simulink model "SPGF_FSK_0000_R2022b"  (R2022b)
settings: Solver=ode4  StartTime=0.0  StopTime=1.4  FixedStep=50e-6/50  RelTol=1e-3  EnableMultiTasking=on
undefined symbols (not defined in the file): D11, Delta
libraries: spsSeriesRLCBranchLib x1646, spsGroundLib x360, spsStairGeneratorLib x147, spsIdealSwitchLib x145, spsCurrentMeasurementLib x145, spsUniversalBridgeLib x76, spsThreePhaseSeriesRLCLoadLib x57, simulink x45, spsBistableLib x36, spsSequenceAnalyzerLib x31, spsThreePhaseParallelRLCLoadLib x20, spsThreePhaseTransformerTwoWindingsLib x20
(part 1 of 40)
settings Model: SimulationMode=accelerator  Creator=Anastasia  LastModifiedBy=Fedot
settings SolverCC: AlgebraicLoopSolver=TrustRegion
settings DataIOCC: SaveFormat=Array  SaveOutput=off  SignalLogging=off  DSMLogging=off  SaveTime=off  ReturnWorkspaceOutputs=off
settings OptimizationCC: BlockReduction=off  OptimizeBlockIOStorage=off  BufferReuse=off  GlobalBufferReuse=off  ExpressionFolding=off  LocalBlockOutputs=off  EfficientMapNaN2IntZero=off  LifeSpan=inf
settings DebuggingCC: UnderspecifiedInitializationDetection=Classic  MergeDetectMultiDrivingBlocksExec=none  SolverPrmCheckMsg=warning  AllowSymbolicDim=off  StateNameClashWarn=warning  SFUnexpectedBacktrackingDiag=warning  SFNoUnconditionalDefaultTransitionDiag=warning  SFExecutionAtInitializationDiag=none  SFMachineParentedDataDiag=warning  ArithmeticOperatorsInVariantConditions=warning
settings HardwareCC: ProdBitPerPointer=32  ProdBitPerSizeT=32  ProdBitPerPtrDiffT=32  ProdLargestAtomicFloat=None  ProdIntDivRoundTo=Undefined  ProdEndianess=Unspecified  ProdWordSize=32  ProdHWDeviceType=32-bit Generic  TargetBitPerPointer=64  TargetBitPerSizeT=64  TargetBitPerPtrDiffT=64  TargetLongLongMode=on  TargetIntDivRoundTo=Zero  TargetEndianess=LittleEndian  TargetWordSize=64  TargetHWDeviceType=MATLAB Host  ProdEqTarget=off
settings ModelReferenceCC: EnableRefExpFcnMdlSchedulingChecks=on  PropagateSignalLabelsOutOfModel=off
settings SFSimCC: SimUseLocalCustomCode=off  CustomCodeUndefinedFunction=UseInterfaceOnly
settings RTWCC: RTWUseLocalCustomCode=off
settings CodeAppCC: MaxIdLength=128  StateflowObjectComments=on
settings GRTTargetCC: TargetLangStandard=C89/C90 (ANSI)  CombineOutputUpdateFcns=off  GRTInterface=on
settings ConfigComp: CovMetricSettings=dw  CovSaveCumulativeToWorkspaceVar=on  CovSaveSingleToWorkspaceVar=on  CovExternalEMLEnable=off
settings SimscapeCC: SimscapeNormalizeSystem=off

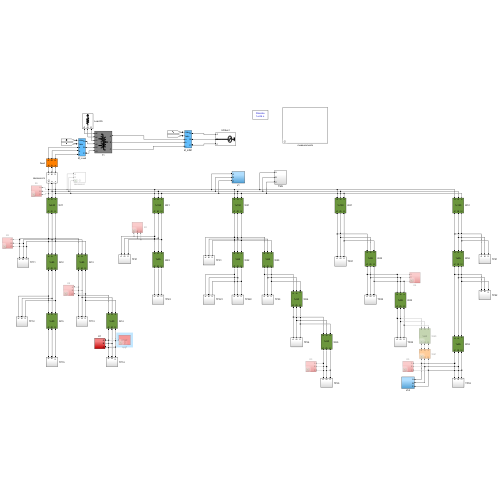
[thumbnail: Simulink's stored preview of the top-level diagram]
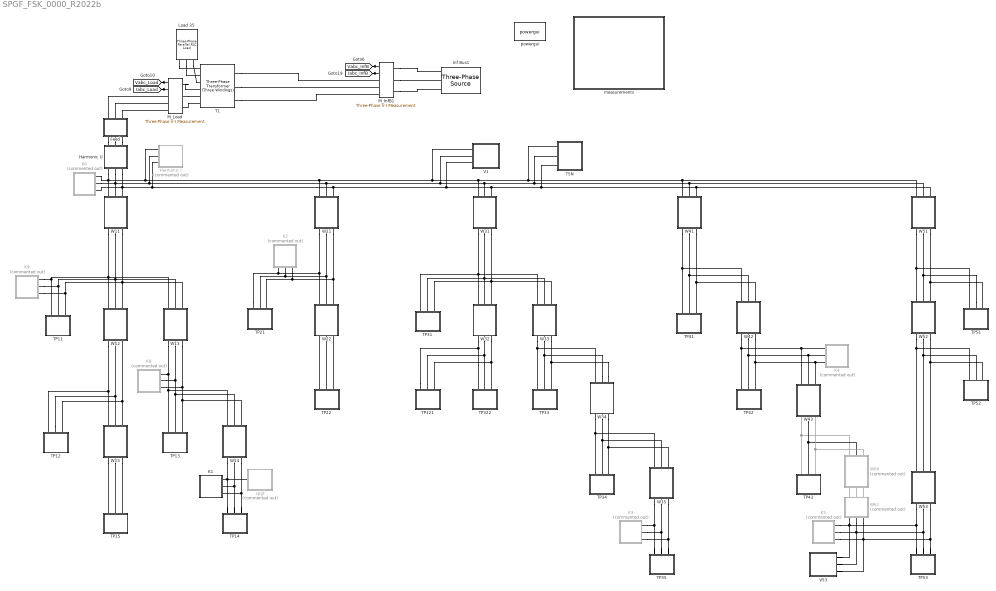
== system SPGF_FSK_0000_R2022b ==
  Feed : Subsystem
      mask Display:
      | port_label('lconn',1,'A');
      | port_label('lconn',2,'B');
      | port_label('lconn',3,'C');
      | 
      | port_label('rconn',1,'a');
      | port_label('rconn',2,'b');
      | port_label('rconn',3,'c');
  Harmonic I : Subsystem  Commented=on  mask(Three-Phase Harmonic Current Source){ActiveABC=[1 0 0], Frequency=50, PhaseABC=[0 -120 120], HN=[5, 7, 11, 13, 17], Current=19.26, Percent=[2.84, 2.42, 1.67, 0.74, 0.3], PhaseH=[0 0 0 0 0]}
      mask prompts: ActiveABC "Active phase of source [A, B, C]"; Frequency "Frequency f [Hz] :"; PhaseABC "Current phase [phA, phB, phC] [degree]"; HN "Vector of harmonic numbers [5, 7, 11, 13 ...] :"; Current "Base current rms [A] :"; Percent "Percent of harmanic in base current [%] :"; PhaseH "Phase of harmonic current [degree] :"
      mask help: Add harmonic to current
      mask init:
      | ActiveA = ActiveABC(1);
      |     ActiveB = ActiveABC(2);
      |     ActiveC = ActiveABC(3);
      |     PhaseA = PhaseABC(1);
      |     PhaseB = PhaseABC(2);
      |     PhaseC = PhaseABC(3);
  Harmonic U : Subsystem  mask(Three-Phase Harmonic Voltage Source){EnableH=off, ActiveABC=[1, 1, 1], Frequency=50, PhaseABC=[0 -120 120], HN=[5, 7, 11, 13, 17], Voltage=1000, Percent=[2.84, 2.42, 1.67, 0.74, 0.3].*1.5, PhaseH=[0 0 0 0 0]}
      mask prompts: EnableH "Enable harmonic voltage source"; ActiveABC "Active phase of source [A, B, C]"; Frequency "Frequency f [Hz] :"; PhaseABC "Voltage phase [phA, phB, phC] [degree]"; HN "Vector of harmonic numbers [5, 7, 11, 13 ...] :"; Voltage "Base Voltage rms [V] :"; Percent "Percent of harmanic in base voltage [%] :"; PhaseH "Phase of harmonic voltage [degree] :"
      mask help:
      | The block allows to add harmonic signals to voltage.
      | The block is connected in series.
      mask init:
      | PhaseA = PhaseABC(1);
      |     PhaseB = PhaseABC(2);
      |     PhaseC = PhaseABC(3);
      |     ActiveA = ActiveABC(1);
      |     ActiveB = ActiveABC(2);
      |     ActiveC = ActiveABC(3);
      mask Callback EnableH:
      | base_block_name = gcb;
      |     enable = get_param(base_block_name, 'EnableH');
      |     if strcmp(enable, 'on')
      |         set_param([base_block_name, '/harmonic'],'Commented','off');
      |         set_param([base_block_name, '/shunt'],'Commented','on');
      |     else
      |         set_param([base_block_name, '/harmonic'],'Commented','on');
      |         set_param([base_block_name, '/shunt'],'Commented','off');
      |     end
  Inf Bus1 : spsThreePhaseSourceLib/Three-Phase Source  InternalConnection=Yg  VoltagePhases=off  Voltage=(115500)*1  PhaseAngle=0  Voltage_phases=[25e3 25e3 25e3]/sqrt(3)  PhaseAngles_phases=[0 -120 +120]  Frequency=50  NonIdealSource=on  SpecifyImpedance=off  Resistance=0  Inductance=0  ShortCircuitLevel=100e6  BaseVoltage=115.5e3  XRratio=7  BusType=swing  Pref=0  Qref=0  Prefabc=[10e3, 10e3, 10e3]  Qrefabc=[0, 0, 0]  Qmin=-inf  Qmax=inf
  K1 : Subsystem
  K2 : Subsystem  Commented=on
  K3 : Subsystem  Commented=on
  K4 : Subsystem  Commented=on
  K5 : Subsystem  Commented=on
  K6 : Subsystem  Commented=on
  K8 : Subsystem  Commented=on
  K9 : Subsystem  Commented=on
  Load 35 : spsThreePhaseParallelRLCLoadLib/Three-Phase Parallel RLC Load  LConnTagsString=A|B|C  Configuration=Y (grounded)  NominalVoltage=(38435.4)*1  Vabc=[1e3 1e3 1e3]  Vabcp=[1e3 1e3 1e3]  NominalFrequency=50  UnbalancedPower=off  ActivePower=1e6  InductivePower=0  CapacitivePower=0  Pabc=[10e3 9e3 11e3]  QLabc=[100 90 110]  QCabc=[100 90 110]  Pabcp=[10e3 9e3 11e3]  QLabcp=[100 90 110]  QCabcp=[100 90 110]  Measurements=None  LoadType=constant PQ
  M_InfB1 : spsThreePhaseVIMeasurementLib/Three-Phase V-I Measurement  VoltageMeasurement=phase-to-ground  SetLabelV=off  LabelV=Vabc  Vpu=off  VpuLL=off  CurrentMeasurement=yes  SetLabelI=off  LabelI=Iabc  Ipu=off  Pbase=100e6  Vbase=500e3  OutputType=Complex  PhasorSimulation=off  PSBequivalent=0
  M_Load : spsThreePhaseVIMeasurementLib/Three-Phase V-I Measurement  VoltageMeasurement=phase-to-ground  SetLabelV=off  LabelV=Vabc  Vpu=off  VpuLL=off  CurrentMeasurement=yes  SetLabelI=off  LabelI=Iabc  Ipu=off  Pbase=100e6  Vbase=500e3  OutputType=Complex  PhasorSimulation=off  PSBequivalent=0
  T1 : spsThreePhaseTransformerThreeWindingsLib/Three-Phase Transformer (Three Windings)  Winding1Connection=Yg  Winding2Connection=Y  Winding3Connection=Delta (D11)  CoreType=Three single-phase transformers  SetSaturation=on  Hysteresis=off  DataFile='hysteresis'  SetInitialFlux=off  Measurements=None  UNITS=pu  NominalPower=[20e6 , 50 ]  Winding1=[115.5e3 , 0.003175 , 0.01025 ]  Winding2=[ 38.5e3 , 0.003175 , -0.0025]  Winding3="[ 11e3 , 0.003175 ,  0.0125 ]"  Rm=444.444  Lm=40  L0=2  Saturation=[0 0;0.01774 0.324129;0.0487637 0.61284;0.0980856 0.825118;0.2 1;0.309543 1.08024;0.652348 1.17344;2.0357 1.26115;6.0215 1.36094;12.4388 1.49469]  InitialFluxes=[-0.996027177222098 0.502063669050136 0.493963508172008]  BreakLoop=on  DiscreteSolver=Trapezoidal iterative  DataType=off  TransfoNumber=1
      settings: LibrarySourceBlock=|
      | sps_lib/Power Grid Elements/Three-Phase
      | Transformer
      | (Three Windings)
  TP11 : Subsystem
  TP12 : Subsystem
  TP13 : Subsystem
  TP14 : Subsystem
  TP15 : Subsystem
  TP21 : Subsystem
  TP22 : Subsystem
  TP31 : Subsystem
  TP321 : Subsystem
  TP322 : Subsystem
  TP33 : Subsystem
  TP34 : Subsystem
  TP35 : Subsystem
  TP41 : Subsystem
  TP42 : Subsystem
  TP43 : Subsystem
  TP51 : Subsystem
  TP52 : Subsystem
  TP53 : Subsystem
  TSN : Subsystem
  V1 : Subsystem
  V53 : Subsystem
  W11 : Subsystem
      mask Display:
      | port_label('lconn',1,'A');
      | port_label('lconn',2,'B');
      | port_label('lconn',3,'C');
      | 
      | port_label('rconn',1,'a');
      | port_label('rconn',2,'b');
      | port_label('rconn',3,'c');
      | disp('1x240');
  W12 : Subsystem
      mask Display:
      | port_label('lconn',1,'A');
      | port_label('lconn',2,'B');
      | port_label('lconn',3,'C');
      | 
      | port_label('rconn',1,'a');
      | port_label('rconn',2,'b');
      | port_label('rconn',3,'c');
      | disp('1x95');
  W13 : Subsystem
      mask Display:
      | port_label('lconn',1,'A');
      | port_label('lconn',2,'B');
      | port_label('lconn',3,'C');
      | 
      | port_label('rconn',1,'a');
      | port_label('rconn',2,'b');
      | port_label('rconn',3,'c');
      | disp('1x95');
  W14 : Subsystem
      mask Display:
      | port_label('lconn',1,'A');
      | port_label('lconn',2,'B');
      | port_label('lconn',3,'C');
      | 
      | port_label('rconn',1,'a');
      | port_label('rconn',2,'b');
      | port_label('rconn',3,'c');
      | disp('1x50');
  W15 : Subsystem
      mask Display:
      | port_label('lconn',1,'A');
      | port_label('lconn',2,'B');
      | port_label('lconn',3,'C');
      | 
      | port_label('rconn',1,'a');
      | port_label('rconn',2,'b');
      | port_label('rconn',3,'c');
      | disp('1x50');
  W21 : Subsystem
      mask Display:
      | port_label('lconn',1,'A');
      | port_label('lconn',2,'B');
      | port_label('lconn',3,'C');
      | 
      | port_label('rconn',1,'a');
      | port_label('rconn',2,'b');
      | port_label('rconn',3,'c');
      | disp('1x150');
  W22 : Subsystem
      mask Display:
      | port_label('lconn',1,'A');
      | port_label('lconn',2,'B');
      | port_label('lconn',3,'C');
      | 
      | port_label('rconn',1,'a');
      | port_label('rconn',2,'b');
      | port_label('rconn',3,'c');
      | disp('1x95');
  W31 : Subsystem
      mask Display:
      | port_label('lconn',1,'A');
      | port_label('lconn',2,'B');
      | port_label('lconn',3,'C');
      | 
      | port_label('rconn',1,'a');
      | port_label('rconn',2,'b');
      | port_label('rconn',3,'c');
      | disp('1x150');
  W32 : Subsystem
      mask Display:
      | port_label('lconn',1,'A');
      | port_label('lconn',2,'B');
      | port_label('lconn',3,'C');
      | 
      | port_label('rconn',1,'a');
      | port_label('rconn',2,'b');
      | port_label('rconn',3,'c');
      | disp('1x95');
  W33 : Subsystem
      mask Display:
      | port_label('lconn',1,'A');
      | port_label('lconn',2,'B');
      | port_label('lconn',3,'C');
      | 
      | port_label('rconn',1,'a');
      | port_label('rconn',2,'b');
      | port_label('rconn',3,'c');
      | disp('1x95');
  W34 : Subsystem
      mask Display:
      | port_label('lconn',1,'A');
      | port_label('lconn',2,'B');
      | port_label('lconn',3,'C');
      | 
      | port_label('rconn',1,'a');
      | port_label('rconn',2,'b');
      | port_label('rconn',3,'c');
      | disp('1x50');
  W35 : Subsystem
      mask Display:
      | port_label('lconn',1,'A');
      | port_label('lconn',2,'B');
      | port_label('lconn',3,'C');
      | 
      | port_label('rconn',1,'a');
      | port_label('rconn',2,'b');
      | port_label('rconn',3,'c');
      | disp('1x50');
  W41 : Subsystem
      mask Display:
      | port_label('lconn',1,'A');
      | port_label('lconn',2,'B');
      | port_label('lconn',3,'C');
      | 
      | port_label('rconn',1,'a');
      | port_label('rconn',2,'b');
      | port_label('rconn',3,'c');
      | disp('1x150');
  W42 : Subsystem
      mask Display:
      | port_label('lconn',1,'A');
      | port_label('lconn',2,'B');
      | port_label('lconn',3,'C');
      | 
      | port_label('rconn',1,'a');
      | port_label('rconn',2,'b');
      | port_label('rconn',3,'c');
      | disp('1x95');
  W43 : Subsystem
      mask Display:
      | port_label('lconn',1,'A');
      | port_label('lconn',2,'B');
      | port_label('lconn',3,'C');
      | 
      | port_label('rconn',1,'a');
      | port_label('rconn',2,'b');
      | port_label('rconn',3,'c');
      | disp('1x95');
  W51 : Subsystem
      mask Display:
      | port_label('lconn',1,'A');
      | port_label('lconn',2,'B');
      | port_label('lconn',3,'C');
      | 
      | port_label('rconn',1,'a');
      | port_label('rconn',2,'b');
      | port_label('rconn',3,'c');
      | disp('1x150');
  W52 : Subsystem
      mask Display:
      | port_label('lconn',1,'A');
      | port_label('lconn',2,'B');
      | port_label('lconn',3,'C');
      | 
      | port_label('rconn',1,'a');
      | port_label('rconn',2,'b');
      | port_label('rconn',3,'c');
      | disp('1x95');
  W53 : Subsystem
      mask Display:
      | port_label('lconn',1,'A');
      | port_label('lconn',2,'B');
      | port_label('lconn',3,'C');
      | 
      | port_label('rconn',1,'a');
      | port_label('rconn',2,'b');
      | port_label('rconn',3,'c');
      | disp('1x95');
  W60 : Subsystem  Commented=on
      mask Display:
      | port_label('lconn',1,'A');
      | port_label('lconn',2,'B');
      | port_label('lconn',3,'C');
      | 
      | port_label('rconn',1,'a');
      | port_label('rconn',2,'b');
      | port_label('rconn',3,'c');
      | disp('1x95');
  W61 : Subsystem  Commented=on
      mask Display:
      | port_label('lconn',1,'A');
      | port_label('lconn',2,'B');
      | port_label('lconn',3,'C');
      | 
      | port_label('rconn',1,'a');
      | port_label('rconn',2,'b');
      | port_label('rconn',3,'c');
  measurements : Subsystem  mask{FTime=0.02/40}
      mask prompts: FTime "Fourier Sample Time"
  powergui : spspowerguiLib/powergui  Priority=1  SimulationMode=Discrete  SampleTime=50e-6/50  frequency=60  Iterations=100  frequencyindice=0  Pbase=1e+06  ErrMax=0.0001  UnitsV=kV  UnitsW=MW  buscounter=0  FunctionMessages=off  echomessages=off  EnableUseOfTLC=off  CurrentSourceSwitches=off  DisableSnubberDevices=off  DisableRonSwitches=off  DisableVfSwitches=off  DisplayEquations=off  AutomaticDiscreteSolvers=off  SolverType=Backward Euler  Interpol=off  ExternalGateDelay=off  methode=off  Ts=0  x0status=blocks  SPID=off  SwTol=0  HookPort=off  NonlinearTolerance=1e-4  nMaxIteration=100  ContinueOnMaxIteration=off  RestoreLinks=warning  ResistiveCurrentMeasurement=off  Frange=[0:2:500]  Ylog=off  Xlog=on  ShowGrid=off  save=off  variable=ZData  structure=0  ZoomFFT=off  StartTime=0.0  cycles=1  DisplayStyle=1  fundamental=60  FreqAxis=off  MaxFrequency=1000  frequencyindicesteady=1  RmsSteady=2  display=off
  spgf : Subsystem  Commented=on  mask(Single Phase-to-Ground Fault (1ph)){FaultResistance=0.0001, GroundResistance=1e-03, SnubberResistance=1e6, SnubberCapacitance=inf, TransitionTimes=[0.2 0.8], InitialPhaseCtrl=off, Freq=50, Units=degrees, FaultDelayDeg=0, FaultDelayRad=0, FaultDelaySec=0, TheoryOfArc=None, WaitTime=0.008, TypeOfArcIgnVoltage=Stair Pattern with Ramp, ArcVoltage=6000, PulseArcVoltage=[6000 600], DurPulseArcVoltage=0.2, SwitchArcVoltage=[6000 600 5000 400], DurArcVoltage=[0.1 0.2 0.1 0.2], EndArcVoltage=[7000 200 5000 900], LimitArcNum=off, ArcingNumber=1, AddTimeDelay=off, TimeDelay=[0 0.1 0.2 ], EnableFilter=off, FreqFilter=200, FilterReturnTime=1e-3, Inter=off, TypeOfPause=None, NoiseSampleTime=0.04, NoiseSeed=23345, PulsePeriod=0.2, PulseWidth=20, PhaseDelay=0, SwitchTimes=[1 1.01 1.2 1.4]}
      mask prompts: FaultResistance "Fault resistance Ron (ohms) :"; GroundResistance "Ground resistance Rg (ohms) :"; SnubberResistance "Snubbers resistance Rp (ohms) :"; SnubberCapacitance "Snubbers capacitance Cp (F) :"; TransitionTimes "Transition times (s) :"; InitialPhaseCtrl "Enable voltage zero crossing control"; Freq "Fundumental frequency (Hz) :"; Units "Units for fault delay"; FaultDelayDeg "Fault delay (Units) :"; FaultDelayRad "Fault delay (Units) :"; FaultDelaySec "Fault delay (Units) :"; TheoryOfArc "Theory of the arcing ground"; WaitTime "Wait time after the arcing (sec):"; TypeOfArcIgnVoltage "Type of Arc Ignition Voltage"; ArcVoltage "Voltage of the arcing (V) :"; PulseArcVoltage "Voltage of the arcing (V) :"; DurPulseArcVoltage "Duration of pulse (sec) :"; SwitchArcVoltage "Voltage of the arcing (V) :"; DurArcVoltage "Duration of Voltage Arc (sec) :"; EndArcVoltage "Voltage of the arcing at the end of each range (V) :"; LimitArcNum "Limit number of arcing [N] :"; ArcingNumber "Number of uprising arcing"; AddTimeDelay "Add time delay :"; TimeDelay "Time delay between arc (sec) [1xN] :"; EnableFilter "Enable lowpass filter"; FreqFilter "Natural frequency of lowpass filter (Hz) [120-250]:"; FilterReturnTime "Filter return time (sec):"; Inter "Interrupt only arc striking"; TypeOfPause "Add pause in the arcing ground"; NoiseSampleTime "Sample time of white noise (s) :"; NoiseSeed "Seed of white noise"; PulsePeriod "Period of pulses (s) :"; PulseWidth "Width of pulse (% of period) :"; PhaseDelay "Phase delay (sec) :"; SwitchTimes "Switch times (sec) [1,0,1,0...] :"
      mask help:
      | The block allows to model single phase-to-groung fault including intermittent arc fault.
      | Two theories of arc extinction, suh as Peterson, Peters and Slepian, are supperted.
      mask init:
      | maskObj = Simulink.Mask.get(gcb);
      |      
      |     % get start time, end time and duration of fault
      |     BeginFaultTime = TransitionTimes(1);
      |     EndFaultTime = TransitionTimes(2);
      |     DurFault = EndFaultTime - BeginFaultTime;
      | 
      |     % Enable Zero Crossing
      |     InitialPhaseCtrl = double(InitialPhaseCtrl);
      | 
      |     % fault delay initialization
      |     units = get_param(gcb,'Units');
      |     FaultDelay = 0;
      |     if strcmp(units, 'degrees')
      |         FaultDelay = FaultDelayDeg / 360 * (1 / Freq);
      |     elseif strcmp(units, 'radians')
      |         FaultDelay = FaultDelayRad / (2*pi) * (1 / Freq);
      |     elseif strcmp(units, 'seconds')
      |         FaultDelay = FaultDelaySec;
      |     end
      |     
      |     % Type of Arc Ignitition Voltage == Linear
      |     Slope = 0;
      |     if (length(ArcVoltage) > 1)
      |         Slope = (ArcVoltage(2)-ArcVoltage(1))/(EndFaultTime-BeginFaultTime);
      |     end
      |     
      |     % Type of Arc Ignitition Voltage == Pulse Generator
      |     VoltageArcBase = PulseArcVoltage(2);
      |     PulseAmpV = PulseArcVoltage(1) - PulseArcVoltage(2);
      |     if (length(DurPulseArcVoltage) == 1)
      |         PulsePeriodV = DurPulseArcVoltage * 2;
      |         PulseWidthV = 50;
      |     else
      |         PulsePeriodV = DurPulseArcVoltage(1) + DurPulseArcVoltage(2);
      |         PulseWidthV = DurPulseArcVoltage(1) / PulsePeriodV * 100;    
      |     end
      |     PulsePhaseDelayV = 0;
      |     
      |     % Type of Arc Ignitition Voltage == Stair Pattern
      |     if (length(SwitchArcVoltage) > length(DurArcVoltage))
      |         j = 1;
      |         for i = length(DurArcVoltage)+1:length(SwitchArcVoltage)
      |             if (j > length(DurArcVoltage))
      |                 j = 1;
      |             end
      |             DurArcVoltage(i) = DurArcVoltage(j);
      |             j = j + 1;
      |         end
      |     end
      |     k =  (DurFault / sum(DurArcVoltage));
      |     if (k > 1)
      |         lengthPattern = fix(k * length(SwitchArcVoltage)) + 1;
      |     else
      |         lengthPattern = length(SwitchArcVoltage);
      |     end
      |     SwitchTimesVoltageArc(1) = BeginFaultTime;
      |     j = 1;
      |     for i=1:lengthPattern
      |         if (j > length(DurArcVoltage))
      |             j = 1;
      |         end   
      |         SwitchTimesVoltageArc(i+1) = SwitchTimesVoltageArc(i) + DurArcVoltage(j);
      |         j = j + 1;
      |     end
      |     j = 1;
      |     AmpVoltageArc = SwitchArcVoltage;
      |     for i=length(SwitchArcVoltage):lengthPattern
      |         AmpVoltageArc(i+1) = SwitchArcVoltage(j);
      |         j = j + 1;
      |     end
      | 
      |     % Type of Arc Ignitition Voltage == Stair Pattern with Ramp
      |     % Ramp settings
      |     j = 1;
      |     for i=length(EndArcVoltage):lengthPattern
      |         EndArcVoltage(i+1) = EndArcVoltage(j);
      |         j = j + 1;
      |     end
      |     j = 1;
      |     DurRampVoltageArc = DurArcVoltage;
      |     for i=length(DurArcVoltage):lengthPattern
      |         DurRampVoltageArc(i+1) = DurRampVoltageArc(j);
      |         j = j + 1;
      |     end
      |     SlopeInPattern = (EndArcVoltage - AmpVoltageArc) ./ DurRampVoltageArc;
      |     
      |     %
      |     SwitchStatus(1) = 0;
      |     for i=1:length(SwitchTimes)
      |         SwitchStatus(i+1) = double(~(logical(SwitchStatus(i))));
      |     end
      |     SwitchTimes = [0,SwitchTimes];
      |     
      |     % Arc Limitation Param
      |     LimitArcNum = double(LimitArcNum);
      |     AddTimeDelay = double(AddTimeDelay);
      |     
      |     if (AddTimeDelay == 0)
      |         TimeDelay = zeros(1,ArcingNumber);
      |     end
      | 
      |     % Enable Filter for detection zero-crossing (Peters & Slepian theory)
      |     EnableFilter = double(EnableFilter);
      |     
      |     % Interruption only arc striking
      |     Inter = double(Inter);
      settings: CloseFcn=|
      | en = get_param(gcb,'MaskEnables');
      | set_param(gcb,'MaskEnables',en)
      | clear enab en;
      settings: MoveFcn=|
      | en = get_param(gcb,'MaskEnables');
      | set_param(gcb,'MaskEnables',en)
      | clear enab en;
      mask Callback InitialPhaseCtrl:
      | maskObj = Simulink.Mask.get(gcb);
      |     enab = get_param(gcb,'InitialPhaseCtrl');
      |     units = get_param(gcb,'Units');
      |     if strcmp(enab,'on')
      |         maskObj.getParameter('Freq').Enabled = 'on';
      |         maskObj.getParameter('Units').Enabled = 'on';
      |         if strcmp(units,'degrees')
      |             maskObj.getParameter('FaultDelayDeg').Enabled = 'on';
      |         elseif strcmp(units,'radians')
      |             maskObj.getParameter('FaultDelayRad').Enabled = 'on';
      |         elseif strcmp(units,'seconds')
      |             maskObj.getParameter('FaultDelaySec').Enabled = 'on';
      |         end
      |     else
      |         maskObj.getParameter('Freq').Enabled = 'off';
      |         maskObj.getParameter('Units').Enabled = 'off';
      |         if strcmp(units,'degrees')
      |             maskObj.getParameter('FaultDelayDeg').Enabled = 'off';
      |         elseif strcmp(units,'radians')
      |             maskObj.getParameter('FaultDelayRad').Enabled = 'off';
      |         elseif strcmp(units,'seconds')
      |             maskObj.getParameter('FaultDelaySec').Enabled = 'off';
      |         end
      |     end
      mask TypeOptions Units: degrees | radians | seconds
      mask Callback Units:
      | maskObj = Simulink.Mask.get(gcb);
      |     units = get_param(gcb,'Units');
      |     if strcmp(units,'degrees')
      |         maskObj.getParameter('FaultDelayDeg').Visible = 'on';
      |         maskObj.getParameter('FaultDelayRad').Visible = 'off';
      |         maskObj.getParameter('FaultDelaySec').Visible = 'off';
      |     elseif strcmp(units,'radians')
      |         maskObj.getParameter('FaultDelayDeg').Visible = 'off';
      |         maskObj.getParameter('FaultDelayRad').Visible = 'on';
      |         maskObj.getParameter('FaultDelaySec').Visible = 'off';
      |     elseif strcmp(units,'seconds')
      |         maskObj.getParameter('FaultDelayDeg').Visible = 'off';
      |         maskObj.getParameter('FaultDelayRad').Visible = 'off';
      |         maskObj.getParameter('FaultDelaySec').Visible = 'on';
      |     end
      mask TypeOptions TheoryOfArc: None | Petersen | Peters & Slepian
      mask Callback TheoryOfArc:
      | maskObj = Simulink.Mask.get(gcb);
      |     param = get_param(gcb,'TheoryOfArc');
      |     if strcmp(param,'None')
      |         maskObj.getDialogControl('ContArcParam').Enabled = 'off';
      |     else
      |         maskObj.getDialogControl('ContArcParam').Enabled = 'on';
      |         if strcmp(param,'Peters & Slepian')
      |             maskObj.getDialogControl('ContFilterPetSlep').Visible = 'on';
      |             maskObj.getDialogControl('ContWaitPetSlep').Visible = 'on';
      |         else
      |             maskObj.getDialogControl('ContFilterPetSlep').Visible = 'off';
      |             maskObj.getDialogControl('ContWaitPetSlep').Visible = 'off';
      |         end
      |     end
      mask TypeOptions TypeOfArcIgnVoltage: Linear | Pulse Generator | Stair Pattern | Stair Pattern with Ramp
      mask Callback TypeOfArcIgnVoltage:
      | maskObj = Simulink.Mask.get(gcb);
      |     param = get_param(gcb,'TypeOfArcIgnVoltage');
      |     if strcmp(param,'Linear')
      |         maskObj.getParameter('ArcVoltage').Visible = 'on';
      |         maskObj.getParameter('PulseArcVoltage').Visible = 'off';
      |         maskObj.getParameter('DurPulseArcVoltage').Visible = 'off';
      |         maskObj.getParameter('SwitchArcVoltage').Visible = 'off';
      |         maskObj.getParameter('DurArcVoltage').Visible = 'off';
      |         maskObj.getParameter('EndArcVoltage').Visible = 'off';
      |     elseif strcmp(param,'Pulse Generator')
      |         maskObj.getParameter('ArcVoltage').Visible = 'off';
      |         maskObj.getParameter('PulseArcVoltage').Visible = 'on';
      |         maskObj.getParameter('DurPulseArcVoltage').Visible = 'on';
      |         maskObj.getParameter('SwitchArcVoltage').Visible = 'off';
      |         maskObj.getParameter('DurArcVoltage').Visible = 'off';
      |         maskObj.getParameter('EndArcVoltage').Visible = 'off';
      |     elseif strcmp(param,'Stair Pattern')
      |         maskObj.getParameter('ArcVoltage').Visible = 'off';
      |         maskObj.getParameter('PulseArcVoltage').Visible = 'off';
      |         maskObj.getParameter('DurPulseArcVoltage').Visible = 'off';
      |         maskObj.getParameter('SwitchArcVoltage').Visible = 'on';
      |         maskObj.getParameter('DurArcVoltage').Visible = 'on';
      |         maskObj.getParameter('EndArcVoltage').Visible = 'off';
      |     elseif strcmp(param,'Stair Pattern with Ramp')
      |         maskObj.getParameter('ArcVoltage').Visible = 'off';
      |         maskObj.getParameter('PulseArcVoltage').Visible = 'off';
      |         maskObj.getParameter('DurPulseArcVoltage').Visible = 'off';
      |         maskObj.getParameter('SwitchArcVoltage').Visible = 'on';
      |         maskObj.getParameter('DurArcVoltage').Visible = 'on';
      |         maskObj.getParameter('EndArcVoltage').Visible = 'on';
      |     end
      mask Callback LimitArcNum:
      | maskObj = Simulink.Mask.get(gcb);
      |     enab = get_param(gcb,'LimitArcNum');
      |     if strcmp(enab,'on')
      |         maskObj.getParameter('ArcingNumber').Visible = 'on';
      |         maskObj.getParameter('AddTimeDelay').Visible = 'on';
      |     else
      |         maskObj.getParameter('ArcingNumber').Visible = 'off';
      |         set_param(gcb,'AddTimeDelay','off');
      |         maskObj.getParameter('AddTimeDelay').Visible = 'off';
      |         maskObj.getParameter('TimeDelay').Visible = 'off';
      |     end
      mask Callback AddTimeDelay:
      | maskObj = Simulink.Mask.get(gcb);
      |     enab = get_param(gcb,'AddTimeDelay');
      |     if strcmp(enab,'on')
      |         maskObj.getParameter('TimeDelay').Visible = 'on';
      |     else
      |         maskObj.getParameter('TimeDelay').Visible = 'off';
      |     end
      mask Callback EnableFilter:
      | maskObj = Simulink.Mask.get(gcb);
      |     enab = get_param(gcb,'EnableFilter');
      |     if strcmp(enab,'on')
      |         maskObj.getParameter('FreqFilter').Visible = 'on';
      |         maskObj.getParameter('FilterReturnTime').Visible = 'on';
      |     else
      |         maskObj.getParameter('FreqFilter').Visible = 'off';
      |         maskObj.getParameter('FilterReturnTime').Visible = 'off';
      |     end
      mask TypeOptions TypeOfPause: None | White Noise | Pulse Generator | Time Dependent Pulses
      mask Callback TypeOfPause:
      | maskObj = Simulink.Mask.get(gcb);
      |     enab = get_param(gcb,'TypeOfPause');
      |     if strcmp(enab,'None')
      |         maskObj.getParameter('NoiseSampleTime').Visible = 'off';
      |         maskObj.getParameter('NoiseSeed').Visible = 'off';
      |         maskObj.getParameter('PulsePeriod').Visible = 'off';
      |         maskObj.getParameter('PulseWidth').Visible = 'off';
      |         maskObj.getParameter('PhaseDelay').Visible = 'off';
      |         maskObj.getParameter('SwitchTimes').Visible = 'off';
      |     elseif strcmp(enab,'White Noise')
      |         maskObj.getParameter('NoiseSampleTime').Visible = 'on';
      |         maskObj.getParameter('NoiseSeed').Visible = 'on';
      |         maskObj.getParameter('PulsePeriod').Visible = 'off';
      |         maskObj.getParameter('PulseWidth').Visible = 'off';
      |         maskObj.getParameter('PhaseDelay').Visible = 'off';
      |         maskObj.getParameter('SwitchTimes').Visible = 'off';
      |     elseif strcmp(enab,'Pulse Generator')
      |         maskObj.getParameter('NoiseSampleTime').Visible = 'off';
      |         maskObj.getParameter('NoiseSeed').Visible = 'off';
      |         maskObj.getParameter('PulsePeriod').Visible = 'on';
      |         maskObj.getParameter('PulseWidth').Visible = 'on';
      |         maskObj.getParameter('PhaseDelay').Visible = 'on';
      |         maskObj.getParameter('SwitchTimes').Visible = 'off';
      |     elseif strcmp(enab,'Time Dependent Pulses')
      |         maskObj.getParameter('NoiseSampleTime').Visible = 'off';
      |         maskObj.getParameter('NoiseSeed').Visible = 'off';
      |         maskObj.getParameter('PulsePeriod').Visible = 'off';
      |         maskObj.getParameter('PulseWidth').Visible = 'off';
      |         maskObj.getParameter('PhaseDelay').Visible = 'off';
      |         maskObj.getParameter('SwitchTimes').Visible = 'on';
      |     end
      mask DialogControl Container4 Prompt: Configuration
      mask DialogControl ContBreakerParam Prompt: Breaker parameters :
      mask DialogControl ContZeroCross Prompt: Control initial voltage phase of first fault
      mask DialogControl Container5 Prompt: Arc Parameters
      mask DialogControl ContArcParam Prompt: Arc fault parameters
      mask DialogControl ContArcVoltage Prompt: Arc Ignition Voltage
      mask DialogControl ContArcLim Prompt: Arc limitations
      mask DialogControl ContFilterPetSlep Prompt: Filtering
      mask DialogControl ContInterruption Prompt: Interruption
      mask DialogControl Container14 Prompt: Settings for different types of fault interruption
      mask Display:
      | % port_label('input',1,'Iabc');
      | 
      | port_label('lconn',1,'');
      | 
      | disp('   SPGF    ');
  tag scope: Iabc_InfB=global, Iabc_Load=global, Vabc_InfB=global, Vabc_Load=global
  wires:
  M_InfB1/1 -> [Vabc_InfB]
  M_InfB1/2 -> [Iabc_InfB]
  M_Load/1 -> [Vabc_Load]
  M_Load/2 -> [Iabc_Load]
  connections:
  M_InfB1/LConn1 -- Inf Bus1/RConn1
  TP12/RConn2 -- W15/RConn2 -- W12/LConn2
  W12/LConn3 -- W15/RConn3 -- TP12/RConn3
  W15/RConn1 -- TP12/RConn1 -- W12/LConn1
  W13/LConn1 -- K8/LConn1 -- W14/RConn1 -- TP13/RConn1
  W13/LConn2 -- K8/LConn2 -- W14/RConn2 -- TP13/RConn2
  W14/RConn3 -- K8/LConn3 -- W13/LConn3 -- TP13/RConn3
  W14/LConn1 -- spgf/LConn1 -- TP14/RConn1 -- K1/LConn1
  K1/LConn2 -- TP14/RConn2 -- W14/LConn2
  TP21/RConn1 -- K2/LConn1 -- W22/RConn1 -- W21/LConn1
  TP21/RConn3 -- K2/LConn3 -- W22/RConn3 -- W21/LConn3
  TP21/RConn2 -- K2/LConn2 -- W22/RConn2 -- W21/LConn2
  W33/RConn2 -- TP31/RConn2 -- W32/RConn2 -- W31/LConn2
  W33/RConn3 -- TP31/RConn3 -- W32/RConn3 -- W31/LConn3
  W33/RConn1 -- TP31/RConn1 -- W32/RConn1 -- W31/LConn1
  TP321/RConn1 -- TP322/RConn1 -- W32/LConn1
  TP321/RConn2 -- TP322/RConn2 -- W32/LConn2
  TP322/RConn3 -- TP321/RConn3 -- W32/LConn3
  W34/RConn3 -- TP33/RConn3 -- W33/LConn3
  W34/RConn1 -- TP33/RConn1 -- W33/LConn1
  W34/RConn2 -- TP33/RConn2 -- W33/LConn2
  W35/RConn3 -- TP34/RConn3 -- W34/LConn3
  W35/RConn1 -- TP34/RConn1 -- W34/LConn1
  W35/RConn2 -- TP34/RConn2 -- W34/LConn2
  TP35/RConn3 -- K3/LConn3 -- W35/LConn3
  TP35/RConn1 -- K3/LConn1 -- W35/LConn1
  TP35/RConn2 -- K3/LConn2 -- W35/LConn2
  W42/RConn2 -- TP41/RConn2 -- W41/LConn2
  W42/RConn1 -- TP41/RConn1 -- W41/LConn1
  W42/RConn3 -- TP41/RConn3 -- W41/LConn3
  W43/RConn3 -- K4/LConn3 -- TP42/RConn3 -- W42/LConn3
  W43/RConn1 -- K4/LConn1 -- TP42/RConn1 -- W42/LConn1
  TP42/RConn2 -- W42/LConn2 -- K4/LConn2 -- W43/RConn2
  W60/RConn1 -- TP43/RConn1 -- W43/LConn1
  TP43/RConn2 -- W60/RConn2 -- W43/LConn2
  W60/RConn3 -- TP43/RConn3 -- W43/LConn3
  W51/LConn3 -- TP51/RConn3 -- W52/RConn3
  W52/RConn1 -- TP51/RConn1 -- W51/LConn1
  TP51/RConn2 -- W51/LConn2 -- W52/RConn2
  TP52/RConn2 -- W53/RConn2 -- W52/LConn2
  TP52/RConn3 -- W53/RConn3 -- W52/LConn3
  TP52/RConn1 -- W53/RConn1 -- W52/LConn1
  T1/LConn2 -- M_InfB1/RConn2
  M_InfB1/LConn2 -- Inf Bus1/RConn2
  Load 35/LConn2 -- T1/RConn2
  M_InfB1/LConn3 -- Inf Bus1/RConn3
  T1/LConn3 -- M_InfB1/RConn3
  T1/LConn1 -- M_InfB1/RConn1
  Load 35/LConn1 -- T1/RConn1
  Load 35/LConn3 -- T1/RConn3
  W15/LConn1 -- TP15/RConn1
  W15/LConn2 -- TP15/RConn2
  TP22/RConn3 -- W22/LConn3
  TP22/RConn1 -- W22/LConn1
  TP22/RConn2 -- W22/LConn2
  W15/LConn3 -- TP15/RConn3
  M_Load/LConn3 -- T1/RConn6
  M_Load/LConn2 -- T1/RConn5
  M_Load/LConn1 -- T1/RConn4
  Feed/LConn1 -- M_Load/RConn1
  Feed/LConn2 -- M_Load/RConn2
  Feed/LConn3 -- M_Load/RConn3
  W14/LConn3 -- TP14/RConn3 -- K1/LConn3
  W11/LConn3 -- K9/LConn3 -- TP11/RConn3 -- W13/RConn3 -- W12/RConn3
  W11/LConn1 -- K9/LConn1 -- TP11/RConn1 -- W13/RConn1 -- W12/RConn1
  W61/LConn2 -- K5/LConn2 -- V53/LConn2 -- TP53/RConn2 -- W53/LConn2
  W61/LConn1 -- K5/LConn1 -- V53/LConn1 -- TP53/RConn1 -- W53/LConn1
  W61/LConn3 -- K5/LConn3 -- V53/LConn3 -- TP53/RConn3 -- W53/LConn3
  Harmonic U/RConn1 -- K6/LConn1 -- W11/RConn1 -- Harmonic I/LConn1 -- W21/RConn1 -- V1/LConn1 -- W31/RConn1 -- TSN/LConn1 -- W51/RConn1 -- W41/RConn1
  Harmonic I/LConn2 -- Harmonic U/RConn2 -- K6/LConn2 -- W11/RConn2 -- W21/RConn2 -- V1/LConn2 -- W51/RConn2 -- W41/RConn2 -- TSN/LConn2 -- W31/RConn2
  TSN/LConn3 -- Harmonic I/LConn3 -- Harmonic U/RConn3 -- W11/RConn3 -- K6/LConn3 -- W21/RConn3 -- V1/LConn3 -- W31/RConn3 -- W51/RConn3 -- W41/RConn3
  W61/RConn1 -- W60/LConn1
  W61/RConn2 -- W60/LConn2
  W61/RConn3 -- W60/LConn3
  TP11/RConn2 -- K9/LConn2 -- W11/LConn2 -- W12/RConn2 -- W13/RConn2
  Feed/RConn1 -- Harmonic U/LConn1
  Feed/RConn2 -- Harmonic U/LConn2
  Feed/RConn3 -- Harmonic U/LConn3

== system SPGF_FSK_0000_R2022b/Feed ==
  Q : Subsystem
  A : PMIOPort  Side=Left
  B : PMIOPort  Port=2  Side=Left
  C : PMIOPort  Port=3  Side=Left
  a : PMIOPort  Port=4  Side=Right
  b : PMIOPort  Port=5  Side=Right
  c : PMIOPort  Port=6  Side=Right
  connections:
  Q/RConn3 -- C/RConn1
  Q/RConn2 -- B/RConn1
  Q/LConn2 -- b/RConn1
  Q/LConn1 -- a/RConn1
  Q/LConn3 -- c/RConn1
  Q/RConn1 -- A/RConn1

== system SPGF_FSK_0000_R2022b/Harmonic I ==
  Clock : Clock
  Constant1 : Constant  Value=PhaseB
  Constant2 : Constant  Value=PhaseC
  Constant3 : Constant  Value=PhaseA
  Constant4 : Constant  Value=ActiveA
  Constant5 : Constant  Value=ActiveB
  Constant6 : Constant  Value=ActiveC
  Ground : spsGroundLib/Ground  LConnTagsString=a
  In A : spsControlledCurrentSourceLib/Controlled Current Source  Initialize=on  Source_Type=AC  Amplitude=0  Phase=0  Frequency=50  Measurements=None
  In B : spsControlledCurrentSourceLib/Controlled Current Source  Initialize=on  Source_Type=AC  Amplitude=0  Phase=-120  Frequency=50  Measurements=None
  In C : spsControlledCurrentSourceLib/Controlled Current Source  Initialize=on  Source_Type=AC  Amplitude=0  Phase=120  Frequency=50  Measurements=None
  Product1 : Product
  Product15 : Product
  Product2 : Product
  R : spsThreePhaseSeriesRLCBranchLib/Three-Phase Series RLC Branch  LConnTagsString=A|B|C  RConnTagsString=A|B|C  BranchType=R  Resistance=1e6  Inductance=0  Capacitance=0  Measurements=None
  Subsystem1 : Subsystem
  Subsystem2 : Subsystem
  Subsystem3 : Subsystem
  Sum of Elements : Sum  Inputs=+
  Sum of Elements1 : Sum  Inputs=+
  Sum of Elements2 : Sum  Inputs=+
  A : PMIOPort  Tag=PMCPort  Side=Left
  B : PMIOPort  Tag=PMCPort  Port=2  Side=Left
  C : PMIOPort  Tag=PMCPort  Port=3  Side=Left
  wires:
  Product2/1 -> In C/1
  Constant6/1 -> Product2/1
  Product1/1 -> In B/1
  Constant5/1 -> Product1/1
  Product15/1 -> In A/1
  Constant4/1 -> Product15/1
  Subsystem3/1(o) -> Sum of Elements/1
  Subsystem1/1(o) -> Sum of Elements1/1
  Subsystem2/1(o) -> Sum of Elements2/1
  Sum of Elements/1 -> Product15/2
  Sum of Elements1/1 -> Product1/2
  Sum of Elements2/1 -> Product2/2
  Constant3/1 -> Subsystem3/2(phase)
  Constant1/1 -> Subsystem1/2(phase)
  Clock/1 -> Subsystem3/1(clock), Subsystem2/1(clock), Subsystem1/1(clock)
  Constant2/1 -> Subsystem2/2(phase)
  connections:
  R/RConn1 -- In A/RConn1
  In B/RConn1 -- R/RConn2
  R/RConn3 -- In C/RConn1
  In C/LConn1 -- Ground/LConn1 -- In A/LConn1 -- In B/LConn1
  B/RConn1 -- R/LConn2
  C/RConn1 -- R/LConn3
  A/RConn1 -- R/LConn1

== system SPGF_FSK_0000_R2022b/Harmonic U ==
  harmonic : Subsystem  Commented=on
  shunt : Subsystem
  A : PMIOPort  Tag=PMCPort  Side=Left
  B : PMIOPort  Tag=PMCPort  Port=2  Side=Left
  C : PMIOPort  Tag=PMCPort  Port=3  Side=Left
  a : PMIOPort  Port=4  Side=Right
  b : PMIOPort  Port=5  Side=Right
  c : PMIOPort  Port=6  Side=Right
  connections:
  harmonic/LConn1 -- shunt/LConn3 -- A/RConn1
  harmonic/RConn3 -- shunt/RConn3 -- c/RConn1
  b/RConn1 -- harmonic/RConn2 -- shunt/RConn2
  a/RConn1 -- harmonic/RConn1 -- shunt/RConn1
  harmonic/LConn3 -- shunt/LConn2 -- C/RConn1
  harmonic/LConn2 -- shunt/LConn1 -- B/RConn1
